simulink model "washout_filter_sim_2020"  (R2020b)
settings: Solver=FixedStepAuto  StartTime=10  StopTime=31.78  FixedStep=0.01  RelTol=1e-3
values from neighbouring files (symbols this model uses):
  arr_ind = 1:1:size(Time,1)    [Init_for_washout_filter.m]
  Cf = 200000    [Init_for_washout_filter.m]    (also in UKF_start.m = 160000)
  Cr = 250000    [Init_for_washout_filter.m]    (also in UKF_start.m = 200000)
  Iz = 3089    [Init_for_washout_filter.m]    (also in UKF_start.m)
  L = 2.941    [Init_for_washout_filter.m]    (also in UKF_start.m)
  lf = 1.65    [Init_for_washout_filter.m]    (also in UKF_start.m)
  lr = L-lf    (= 1.291)    [Init_for_washout_filter.m]    (also in UKF_start.m)
  mass = 2010.5    [Init_for_washout_filter.m]    (also in UKF_start.m)
  Ratio = 16.3    [Init_for_washout_filter.m]    (also in UKF_start.m)
  rollGrad = 4.5    [Init_for_washout_filter.m]    (also in UKF_start.m)
  rx = 0.29    [Init_for_washout_filter.m]    (also in UKF_start.m = -0.29)
  ry = 0    [Init_for_washout_filter.m]    (also in UKF_start.m)
  T = 0.8    [Init_for_washout_filter.m]
  Time = vbo.channels(1, 2).data-vbo.channels(1, 2).data(1,1)    [Init_for_washout_filter.m]    (also in UKF_start.m)
  Ts = 0.01    [Init_for_washout_filter.m]    (also in UKF_start.m)
undefined symbols (not defined in the file or in its folder): a, b, c, T_var
libraries: cstblocks x2, hdlsllib x1, ctrlSharedLib x1, simulink_extras x1
settings Model: Creator=tawsi_000  LastModifiedBy=rivaa
settings DebuggingCC: UnconnectedInputMsg=none  UnconnectedOutputMsg=none  UnconnectedLineMsg=none  SFMachineParentedDataDiag=error
settings ModelReferenceCC: EnableRefExpFcnMdlSchedulingChecks=off

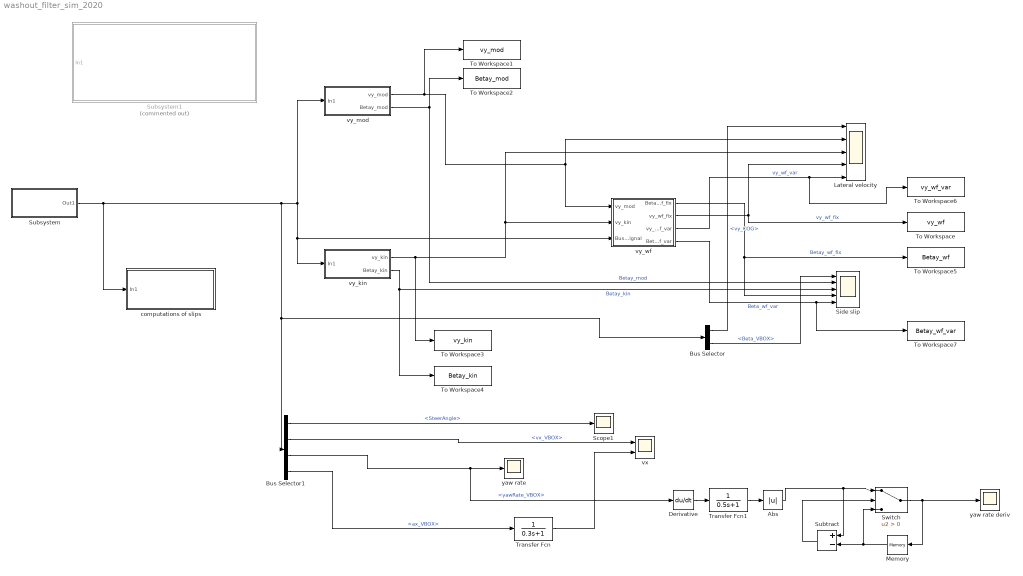
== system washout_filter_sim_2020 ==
  Abs : Abs
  Bus Selector : BusSelector  OutputSignals=vy_COG,Beta_VBOX
  Bus Selector1 : BusSelector  OutputSignals=SteerAngle,vx_VBOX,yawRate_VBOX,ax_VBOX
  Derivative : Derivative
  Lateral velocity : Scope  NumInputPorts=5
  Memory : Memory
  Scope1 : Scope
  Side slip : Scope  NumInputPorts=5
  Subsystem : Subsystem
  Subsystem1 : Subsystem  Commented=on
  Subtract : Sum  Inputs=+-
  Switch : Switch  Criteria=u2 > Threshold
  To Workspace : ToWorkspace  VariableName=vy_wf  SaveFormat=Timeseries  SampleTime=-1
  To Workspace1 : ToWorkspace  VariableName=vy_mod  SaveFormat=Timeseries  SampleTime=-1
  To Workspace2 : ToWorkspace  VariableName=Betay_mod  SaveFormat=Timeseries  SampleTime=-1
  To Workspace3 : ToWorkspace  VariableName=vy_kin  SaveFormat=Timeseries  SampleTime=-1
  To Workspace4 : ToWorkspace  VariableName=Betay_kin  SaveFormat=Timeseries  SampleTime=-1
  To Workspace5 : ToWorkspace  VariableName=Betay_wf  SaveFormat=Timeseries  SampleTime=-1
  To Workspace6 : ToWorkspace  VariableName=vy_wf_var  SaveFormat=Timeseries  SampleTime=-1
  To Workspace7 : ToWorkspace  VariableName=Betay_wf_var  SaveFormat=Timeseries  SampleTime=-1
  Transfer Fcn : TransferFcn  Denominator=[0.3 1]
  Transfer Fcn1 : TransferFcn  Denominator=[0.5 1]
  computations of slips : Subsystem
  vx : Scope  NumInputPorts=2
  vy_kin : Subsystem
  vy_mod : Subsystem
  vy_wf : Subsystem
  yaw rate : Scope
  yaw rate deriv : Scope
  wires:
  vy_wf/2(vy_wf_fix) -> To Workspace/1, Lateral velocity/4  "vy_wf_fix"
  Subsystem/1(Out1) -> computations of slips/1(In1), Bus Selector1/1, Bus Selector/1, vy_kin/1(In1), vy_wf/3(Bus signal), vy_mod/1(In1)
  vy_mod/2(Betay_mod) -> To Workspace2/1, Side slip/2  "Betay_mod"
  vy_kin/2(Betay_kin) -> To Workspace4/1, Side slip/3  "Betay_kin"
  vy_mod/1(vy_mod) -> To Workspace1/1, Lateral velocity/2, vy_wf/1(vy_mod)
  vy_kin/1(vy_kin) -> To Workspace3/1, Lateral velocity/3, vy_wf/2(vy_kin)
  vy_wf/1(Betay_wf_fix) -> Side slip/4, To Workspace5/1  "Betay_wf_fix"
  Bus Selector/2 -> Side slip/1  "<Beta_VBOX>"
  Bus Selector/1 -> Lateral velocity/1  "<vy_COG>"
  Bus Selector1/1 -> Scope1/1  "<SteerAngle>"
  Bus Selector1/2 -> vx/1  "<vx_VBOX>"
  Bus Selector1/3 -> Derivative/1, yaw rate/1  "<yawRate_VBOX>"
  vy_wf/4(Bet_wf_var) -> To Workspace7/1, Side slip/5  "Beta_wf_var"
  vy_wf/3(vy_wf_var) -> To Workspace6/1, Lateral velocity/5  "vy_wf_var"
  Bus Selector1/4 -> Transfer Fcn/1  "<ax_VBOX>"
  Transfer Fcn/1 -> vx/2
  Derivative/1 -> Transfer Fcn1/1
  Abs/1 -> Subtract/1, Switch/1
  Transfer Fcn1/1 -> Abs/1
  Switch/1 -> yaw rate deriv/1, Memory/1
  Memory/1 -> Switch/3, Subtract/2
  Subtract/1 -> Switch/2

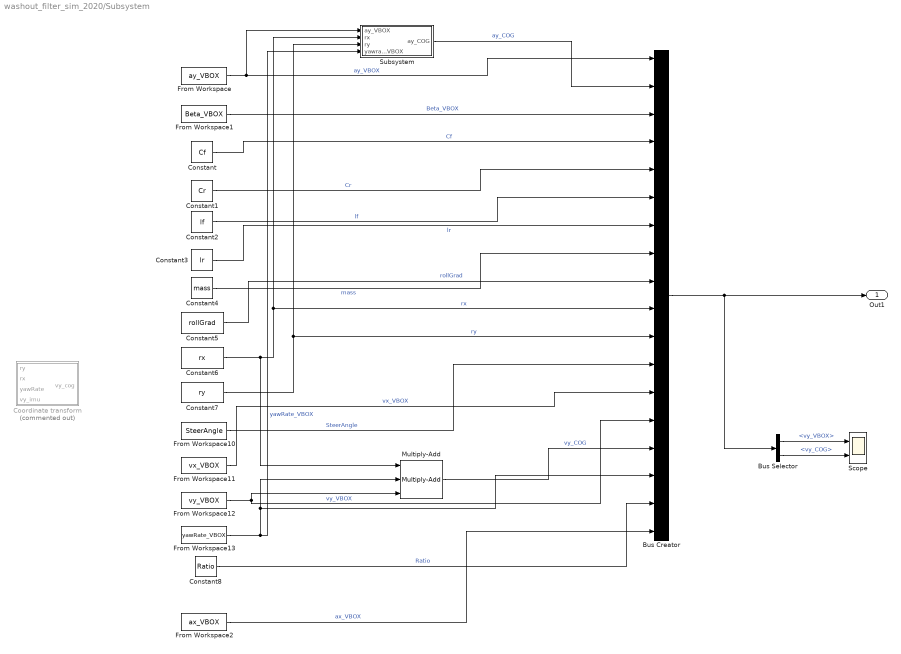
== system washout_filter_sim_2020/Subsystem ==
  Bus Creator : BusCreator  Inputs=18
  Bus Selector : BusSelector  OutputSignals=vy_VBOX,vy_COG
  Constant : Constant  Value=Cf
  Constant1 : Constant  Value=Cr
  Constant2 : Constant  Value=lf
  Constant3 : Constant  Value=lr
  Constant4 : Constant  Value=mass
  Constant5 : Constant  Value=rollGrad
  Constant6 : Constant  Value=rx
  Constant7 : Constant  Value=ry
  Constant8 : Constant  Value=Ratio
  Coordinate transform : MATLAB Function  Commented=on  TreatAsAtomicUnit=on
  From Workspace : FromWorkspace  VariableName=ay_VBOX  SampleTime=Ts
  From Workspace1 : FromWorkspace  VariableName=Beta_VBOX  SampleTime=Ts
  From Workspace10 : FromWorkspace  VariableName=SteerAngle  SampleTime=Ts
  From Workspace11 : FromWorkspace  VariableName=vx_VBOX  SampleTime=Ts
  From Workspace12 : FromWorkspace  VariableName=vy_VBOX  SampleTime=Ts
  From Workspace13 : FromWorkspace  VariableName=yawRate_VBOX  SampleTime=Ts
  From Workspace2 : FromWorkspace  VariableName=ax_VBOX
  Multiply-Add : hdlsllib/HDL Operations/Multiply-Add  Function=c+(a.*b)  datatype=Inherit: Inherit via internal rule  DoSatur=off  FMA=off
      settings: SourceProductBaseCode=SL
  Scope : Scope  NumInputPorts=2
  Subsystem : Subsystem
  Out1 : Outport
  wires:
  From Workspace/1 -> Subsystem/1(ay_VBOX), Bus Creator/1  "ay_VBOX"
  From Workspace1/1 -> Bus Creator/3  "Beta_VBOX"
  Constant/1 -> Bus Creator/4  "Cf"
  Constant1/1 -> Bus Creator/5  "Cr"
  Constant2/1 -> Bus Creator/6  "lf"
  Constant3/1 -> Bus Creator/7  "lr"
  Bus Creator/1 -> Bus Selector/1, Out1/1
  Constant4/1 -> Bus Creator/8  "mass"
  Constant5/1 -> Bus Creator/9  "rollGrad"
  From Workspace12/1 -> Multiply-Add/3, Bus Creator/14  "vy_VBOX"
  Constant6/1 -> Multiply-Add/1, Subsystem/2(rx), Bus Creator/10  "rx"
  From Workspace13/1 -> Subsystem/4(yawrate_VBOX), Multiply-Add/2, Bus Creator/16  "yawRate_VBOX"
  Constant7/1 -> Subsystem/3(ry), Bus Creator/11  "ry"
  From Workspace10/1 -> Bus Creator/12  "SteerAngle"
  From Workspace11/1 -> Bus Creator/13  "vx_VBOX"
  Multiply-Add/1 -> Bus Creator/15  "vy_COG"
  Subsystem/1(ay_COG) -> Bus Creator/2  "ay_COG"
  Constant8/1 -> Bus Creator/17  "Ratio"
  From Workspace2/1 -> Bus Creator/18  "ax_VBOX"
  Bus Selector/1 -> Scope/1  "<vy_VBOX>"
  Bus Selector/2 -> Scope/2  "<vy_COG>"

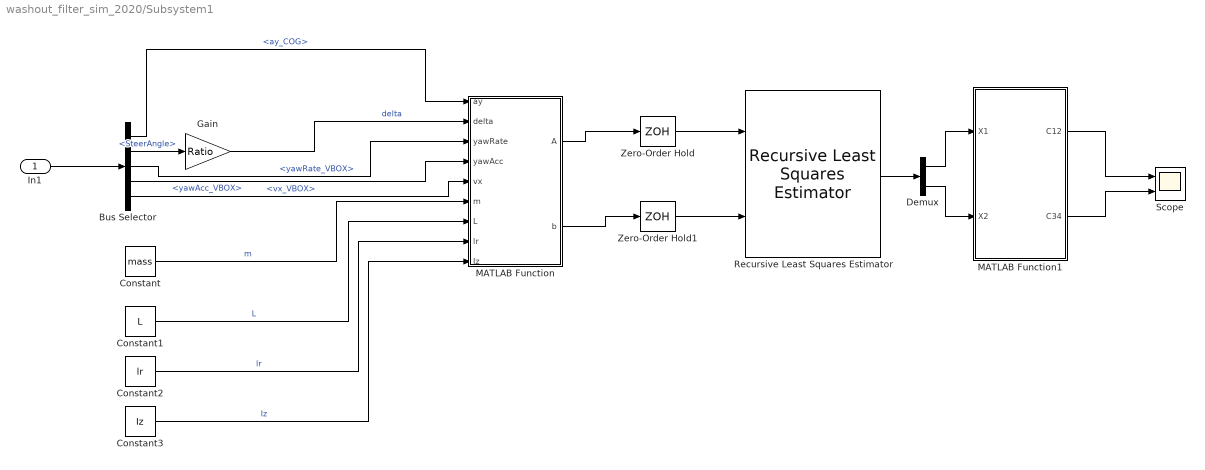
== system washout_filter_sim_2020/Subsystem1 ==
  In1 : Inport
  Bus Selector : BusSelector  OutputSignals=ay_COG,SteerAngle,yawRate_VBOX,yawAcc_VBOX,vx_VBOX
  Constant : Constant  Value=mass
  Constant1 : Constant  Value=L
  Constant2 : Constant  Value=lr
  Constant3 : Constant  Value=Iz
  Demux : Demux  Outputs=2
  Gain : Gain  Gain=Ratio
  MATLAB Function : MATLAB Function  TreatAsAtomicUnit=on
  MATLAB Function1 : MATLAB Function  TreatAsAtomicUnit=on
  Recursive Least Squares Estimator : ctrlSharedLib/Recursive Least Squares Estimator  InitialEstimateSource=None  InitialParameterData=2  P0=1e4  InitialRegressors=0  InitialOutputs=0  History=Infinite  WindowLength=200  EstimationMethod=Forgetting Factor  AdaptationParameter=1  HasTimeVaryingAdaptationParameter=off  NormalizationBias=eps  OutputError=off  OutputP=off  AddEnablePort=off  InputProcessing=Sample-based  Ts=-1
      settings: SourceProductBaseCode=CT,ID
  Scope : Scope  NumInputPorts=2
  Zero-Order Hold : ZeroOrderHold  SampleTime=0.01
  Zero-Order Hold1 : ZeroOrderHold  SampleTime=0.01
  wires:
  In1/1 -> Bus Selector/1
  Bus Selector/2 -> Gain/1  "<SteerAngle>"
  Gain/1 -> MATLAB Function/2(delta)  "delta"
  Bus Selector/3 -> MATLAB Function/3(yawRate)  "<yawRate_VBOX>"
  Constant1/1 -> MATLAB Function/7(L)  "L"
  Constant/1 -> MATLAB Function/6(m)  "m"
  Bus Selector/1 -> MATLAB Function/1(ay)  "<ay_COG>"
  Bus Selector/5 -> MATLAB Function/5(vx)  "<vx_VBOX>"
  Constant2/1 -> MATLAB Function/8(lr)  "lr"
  Constant3/1 -> MATLAB Function/9(Iz)  "Iz"
  MATLAB Function/2(b) -> Zero-Order Hold1/1
  MATLAB Function/1(A) -> Zero-Order Hold/1
  Recursive Least Squares Estimator/1 -> Demux/1
  Demux/1 -> MATLAB Function1/1(X1)
  Demux/2 -> MATLAB Function1/2(X2)
  MATLAB Function1/1(C12) -> Scope/1
  MATLAB Function1/2(C34) -> Scope/2
  Zero-Order Hold1/1 -> Recursive Least Squares Estimator/2
  Zero-Order Hold/1 -> Recursive Least Squares Estimator/1
  Bus Selector/4 -> MATLAB Function/4(yawAcc)  "<yawAcc_VBOX>"

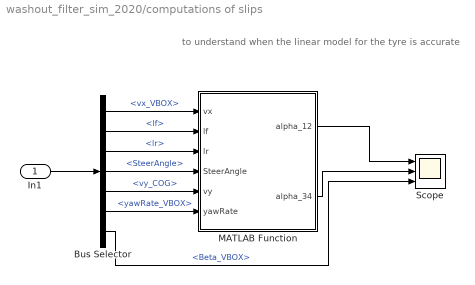
== system washout_filter_sim_2020/computations of slips ==
  note: to understand when the linear model for the tyre is accurate
  In1 : Inport
  Bus Selector : BusSelector  OutputSignals=vx_VBOX,lf,lr,SteerAngle,vy_COG,yawRate_VBOX,Beta_VBOX
  MATLAB Function : MATLAB Function  TreatAsAtomicUnit=on
  Scope : Scope  NumInputPorts=3
  wires:
  In1/1 -> Bus Selector/1
  Bus Selector/1 -> MATLAB Function/1(vx)  "<vx_VBOX>"
  Bus Selector/2 -> MATLAB Function/2(lf)  "<lf>"
  Bus Selector/3 -> MATLAB Function/3(lr)  "<lr>"
  Bus Selector/4 -> MATLAB Function/4(SteerAngle)  "<SteerAngle>"
  Bus Selector/5 -> MATLAB Function/5(vy)  "<vy_COG>"
  Bus Selector/6 -> MATLAB Function/6(yawRate)  "<yawRate_VBOX>"
  MATLAB Function/1(alpha_12) -> Scope/1
  MATLAB Function/2(alpha_34) -> Scope/2
  Bus Selector/7 -> Scope/3  "<Beta_VBOX>"

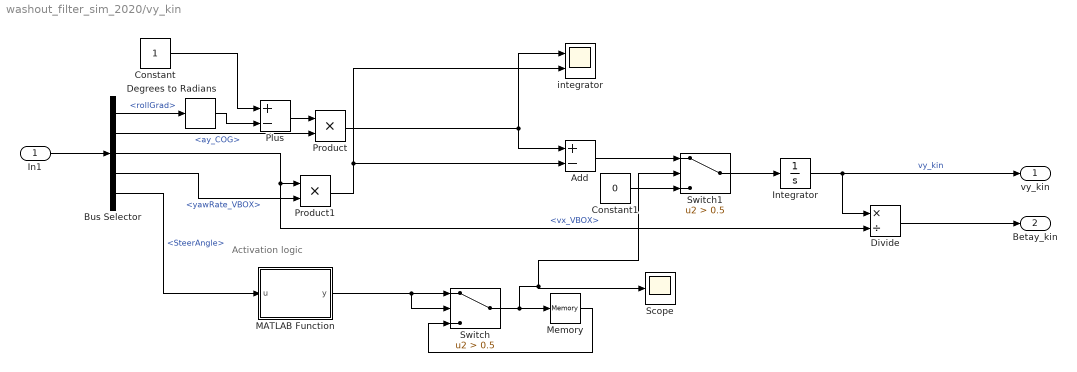
== system washout_filter_sim_2020/vy_kin ==
  note: Activation logic
  In1 : Inport
  Add : Sum  Inputs=+-
  Bus Selector : BusSelector  OutputSignals=rollGrad,ay_COG,vx_VBOX,yawRate_VBOX,SteerAngle
  Constant : Constant
  Constant1 : Constant  Value=0
  Degrees to Radians : simulink_extras/Transformations/Degrees to Radians
  Divide : Product  Inputs=*/
  Integrator : Integrator
  MATLAB Function : MATLAB Function  TreatAsAtomicUnit=on
  Memory : Memory
  Plus : Sum  Inputs=+-
  Product : Product
  Product1 : Product
  Scope : Scope
  Switch : Switch  Criteria=u2 > Threshold  Threshold=0.5
  Switch1 : Switch  Criteria=u2 > Threshold  Threshold=0.5
  integrator : Scope  NumInputPorts=2
  vy_kin : Outport
  Betay_kin : Outport  Port=2
  wires:
  Bus Selector/5 -> MATLAB Function/1(u)  "<SteerAngle>"
  Bus Selector/4 -> Product1/2  "<yawRate_VBOX>"
  MATLAB Function/1(y) -> Switch/2, Switch/1
  Product/1 -> integrator/1, Add/1
  Bus Selector/2 -> Product/2  "<ay_COG>"
  Constant/1 -> Plus/1
  Divide/1 -> Betay_kin/1
  Degrees to Radians/1 -> Plus/2
  Bus Selector/3 -> Divide/2, Product1/1  "<vx_VBOX>"
  Plus/1 -> Product/1
  Memory/1 -> Switch/3
  Bus Selector/1 -> Degrees to Radians/1  "<rollGrad>"
  Product1/1 -> Add/2, integrator/2
  Switch/1 -> Switch1/2, Scope/1, Memory/1
  Integrator/1 -> vy_kin/1, Divide/1  "vy_kin"
  In1/1 -> Bus Selector/1
  Constant1/1 -> Switch1/3
  Add/1 -> Switch1/1
  Switch1/1 -> Integrator/1

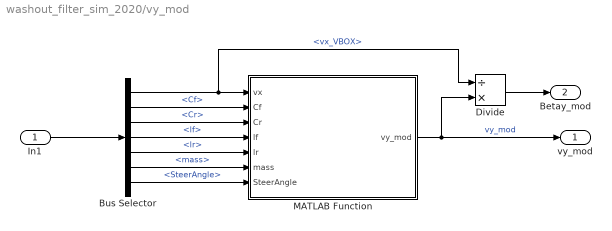
== system washout_filter_sim_2020/vy_mod ==
  In1 : Inport
  Bus Selector : BusSelector  OutputSignals=vx_VBOX,Cf,Cr,lf,lr,mass,SteerAngle
  Divide : Product  Inputs=/*
  MATLAB Function : MATLAB Function  TreatAsAtomicUnit=on
  vy_mod : Outport
  Betay_mod : Outport  Port=2
  wires:
  In1/1 -> Bus Selector/1
  Bus Selector/1 -> Divide/1, MATLAB Function/1(vx)  "<vx_VBOX>"
  Bus Selector/2 -> MATLAB Function/2(Cf)  "<Cf>"
  Bus Selector/3 -> MATLAB Function/3(Cr)  "<Cr>"
  Bus Selector/4 -> MATLAB Function/4(lf)  "<lf>"
  Bus Selector/5 -> MATLAB Function/5(lr)  "<lr>"
  Bus Selector/6 -> MATLAB Function/6(mass)  "<mass>"
  Bus Selector/7 -> MATLAB Function/7(SteerAngle)  "<SteerAngle>"
  MATLAB Function/1(vy_mod) -> Divide/2, vy_mod/1  "vy_mod"
  Divide/1 -> Betay_mod/1

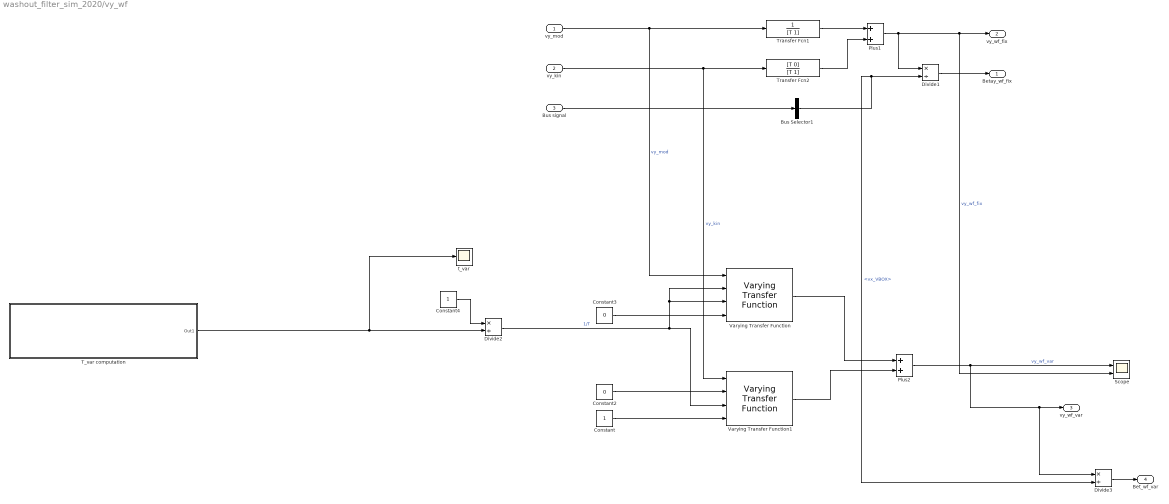
== system washout_filter_sim_2020/vy_wf ==
  vy_mod : Inport
  vy_kin : Inport  Port=2
  Bus signal : Inport  Port=3
  Bus Selector1 : BusSelector  OutputSignals=vx_VBOX
  Constant : Constant
  Constant2 : Constant  Value=0
  Constant3 : Constant  Value=0
  Constant4 : Constant
  Divide1 : Product  Inputs=*/
  Divide2 : Product  Inputs=*/
  Divide3 : Product  Inputs=*/
  Plus1 : Sum
  Plus2 : Sum
  Scope : Scope  NumInputPorts=2
  T_var computation : Subsystem
  Transfer Fcn1 : TransferFcn  Denominator=[T 1]
  Transfer Fcn2 : TransferFcn  Numerator=[T 0]  Denominator=[T 1]
  Varying Transfer Function : cstblocks/Linear Parameter Varying/Varying Transfer Function  N=1
  Varying Transfer Function1 : cstblocks/Linear Parameter Varying/Varying Transfer Function  N=1
  t_var : Scope
  Betay_wf_fix : Outport
  vy_wf_fix : Outport  Port=2
  vy_wf_var : Outport  Port=3
  Bet_wf_var : Outport  Port=4
  wires:
  vy_mod/1 -> Transfer Fcn1/1, Varying Transfer Function/1  "vy_mod"
  vy_kin/1 -> Varying Transfer Function1/1, Transfer Fcn2/1  "vy_kin"
  Transfer Fcn1/1 -> Plus1/1
  Transfer Fcn2/1 -> Plus1/2
  Bus Selector1/1 -> Divide1/2, Divide3/2  "<vx_VBOX>"
  Divide1/1 -> Betay_wf_fix/1
  Bus signal/1 -> Bus Selector1/1
  Plus1/1 -> Scope/2, vy_wf_fix/1, Divide1/1  "vy_wf_fix"
  Varying Transfer Function1/1 -> Plus2/2
  Varying Transfer Function/1 -> Plus2/1
  Constant4/1 -> Divide2/1
  Divide2/1 -> Varying Transfer Function1/3, Varying Transfer Function/3, Varying Transfer Function/2  "1/T"
  Constant3/1 -> Varying Transfer Function/4
  Constant/1 -> Varying Transfer Function1/4
  Constant2/1 -> Varying Transfer Function1/2
  T_var computation/1(Out1) -> t_var/1, Divide2/2
  Plus2/1 -> Divide3/1, vy_wf_var/1, Scope/1  "vy_wf_var"
  Divide3/1 -> Bet_wf_var/1

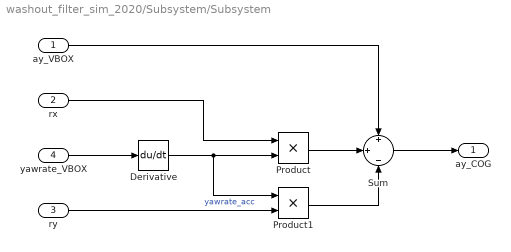
== system washout_filter_sim_2020/Subsystem/Subsystem ==
  ay_VBOX : Inport
  rx : Inport  Port=2
  ry : Inport  Port=3
  yawrate_VBOX : Inport  Port=4
  Derivative : Derivative
  Product : Product
  Product1 : Product
  Sum : Sum  Inputs=+|+|-
  ay_COG : Outport
  wires:
  yawrate_VBOX/1 -> Derivative/1
  Derivative/1 -> Product1/1, Product/2  "yawrate_acc"
  rx/1 -> Product/1
  ry/1 -> Product1/2
  Product/1 -> Sum/2
  ay_VBOX/1 -> Sum/1
  Product1/1 -> Sum/3
  Sum/1 -> ay_COG/1

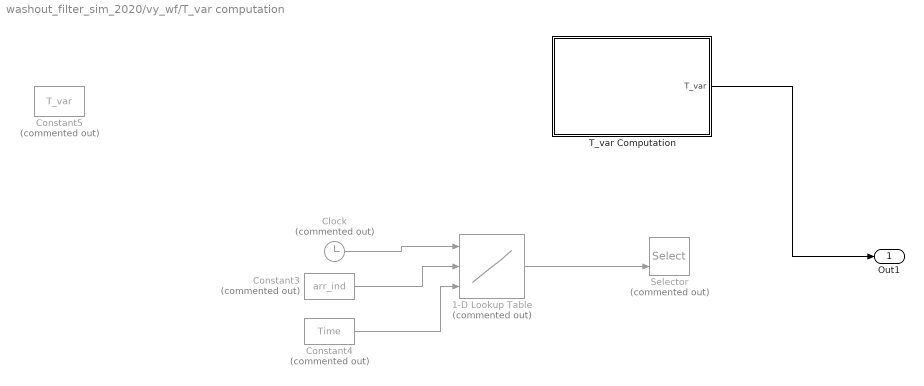
== system washout_filter_sim_2020/vy_wf/T_var computation ==
  1-D Lookup Table : Lookup_n-D  Commented=on  NumberOfTableDimensions=1  BreakpointsForDimension1Source=Input port  BreakpointsForDimension1=Time(1):0.01:Time(end)  TableSource=Input port  Table=1:1:size(Time,1)  InternalRulePriority=Speed  RndMeth=Simplest  InputSameDT=on
      settings: InputPortMap=u0,p221,p5
  Clock : Clock  Commented=on
  Constant3 : Constant  Commented=on  Value=arr_ind
  Constant4 : Constant  Commented=on  Value=Time
  Constant5 : Constant  Commented=on  Value=T_var
  Selector : Selector  Commented=on  InputPortWidth=size(T_var,1)  IndexOptions=Index vector (port)  Indices=[1 3]  OutputSizes=1
  T_var Computation : Subsystem
  Out1 : Outport
  wires:
  Constant3/1 -> 1-D Lookup Table/2
  Constant4/1 -> 1-D Lookup Table/3
  1-D Lookup Table/1 -> Selector/2
  ? -> Selector/1
  Clock/1 -> 1-D Lookup Table/1
  T_var Computation/1(T_var) -> Out1/1

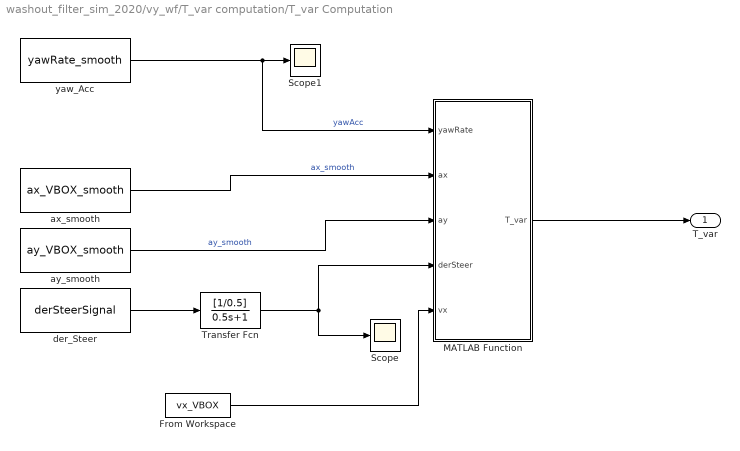
== system washout_filter_sim_2020/vy_wf/T_var computation/T_var Computation ==
  From Workspace : FromWorkspace  VariableName=vx_VBOX
  MATLAB Function : MATLAB Function  TreatAsAtomicUnit=on
  Scope : Scope
  Scope1 : Scope
  Transfer Fcn : TransferFcn  Numerator=[1/0.5]  Denominator=[0.5 1]
  ax_smooth : FromWorkspace  VariableName=ax_VBOX_smooth
  ay_smooth : FromWorkspace  VariableName=ay_VBOX_smooth
  der_Steer : FromWorkspace  VariableName=derSteerSignal
  yaw_Acc : FromWorkspace  VariableName=yawRate_smooth
  T_var : Outport
  wires:
  der_Steer/1 -> Transfer Fcn/1
  ax_smooth/1 -> MATLAB Function/2(ax)  "ax_smooth"
  ay_smooth/1 -> MATLAB Function/3(ay)  "ay_smooth"
  MATLAB Function/1(T_var) -> T_var/1
  Transfer Fcn/1 -> MATLAB Function/4(derSteer), Scope/1
  yaw_Acc/1 -> MATLAB Function/1(yawRate), Scope1/1  "yawAcc"
  From Workspace/1 -> MATLAB Function/5(vx)

== matlab function washout_filter_sim_2020/vy_kin/MATLAB Function ==
  data: u input; y output
function y = fcn(u)

if abs(u)>0.03
    y=1;
else
    y=0;
end

== matlab function washout_filter_sim_2020/vy_mod/MATLAB Function ==
  data: vx input; vy_mod output; Cf input; Cr input; lf input; lr input; mass input; SteerAngle input
function vy_mod = fcn(vx, Cf, Cr, lf, lr, mass, SteerAngle)

vy_mod = SteerAngle*(vx.*(lr*Cf*Cr*(lf+lr)-lf*Cf*mass*(vx.^2)))...
    /((lf+lr)^2*Cf*Cr+mass*(vx.^2)*(lr*Cr-lf*Cf));

== matlab function washout_filter_sim_2020/Subsystem/Coordinate transform ==
  data: ry input; rx input; yawRate input; vy_imu input; vy_cog output
function vy_cog = fcn(ry,rx,yawRate,vy_imu)
    
vy_cog = vy_imu + rx.*yawRate-ry.*yawRate;

== matlab function washout_filter_sim_2020/Subsystem1/MATLAB Function ==
  data: ay input; delta input; yawRate input; yawAcc input; vx input; m input; A output; L input; lr input; Iz input; b output
function [A,b] = fcn(ay,delta,yawRate,yawAcc,vx,m,L,lr,Iz)
 A = [m*L.*ay, L*(delta- L.*yawRate./vx)];
 b = Iz.*yawAcc+m*lr.*ay;

== matlab function washout_filter_sim_2020/Subsystem1/MATLAB Function1 ==
  data: X1 input; X2 input; C12 output; C34 output
function [C12,C34] = fcn(X1,X2)
 C34 = X2./X1;
 C12 = (X1./(1-X1)).*C34;

== matlab function washout_filter_sim_2020/vy_wf/T_var computation/T_var Computation/MATLAB Function ==
  data: yawRate input; ax input; T_var output; ay input; derSteer input; vx input
function T_var = fcn(yawRate, ax,ay,derSteer, vx)

%T_var = min(inf,max(0.01,0.5*abs(yawRate)+0.01*vx)); %sim3 not much
%improved
T_var = min(inf,max(0.01,abs(yawRate)+1.5*abs(ax)));

== matlab function washout_filter_sim_2020/computations of slips/MATLAB Function ==
  data: vx input; alpha_12 output; lf input; lr input; SteerAngle input; vy input; yawRate input; alpha_34 output
function [alpha_12,alpha_34] = fcn(vx,lf,lr,SteerAngle,vy,yawRate)
alpha_12 = atan2((vy+yawRate*lf),vx)-SteerAngle;
alpha_34 = atan2((vy-yawRate*lr),vx);
